simulink model "qhug_9"  (R2021a)
settings: Solver=ode45  StartTime=0.0  StopTime=1700  FixedStep=1  MaxStep=0.01  RelTol=1e-3
settings Model: Creator=daoist  LastModifiedBy=daoist

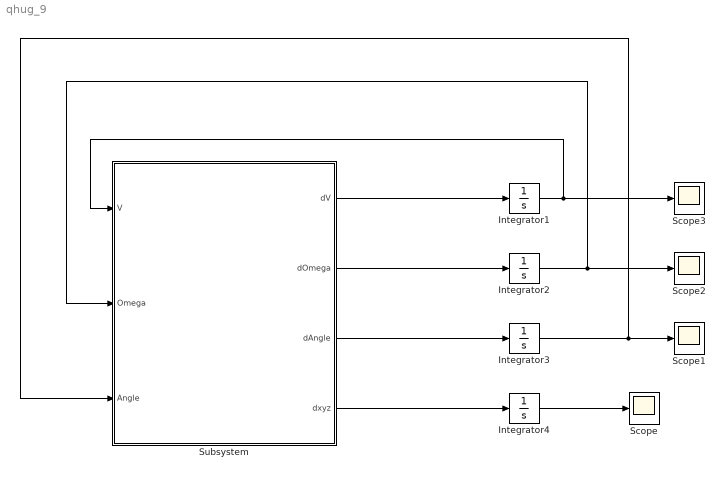
== system qhug_9 ==
  Integrator1 : Integrator  InitialCondition=[0.01 0 0 ]  LimitOutput=on  UpperSaturationLimit=[0.35 0.05 0.01]  LowerSaturationLimit=-[0.35 0.05 0.01]
  Integrator2 : Integrator
  Integrator3 : Integrator
  Integrator4 : Integrator
  Scope{,1..3} (4 alike) : Scope
  Subsystem : Subsystem
  wires:
  Subsystem/1(dV) -> Integrator1/1
  Subsystem/2(dOmega) -> Integrator2/1
  Subsystem/3(dAngle) -> Integrator3/1
  Subsystem/4(dxyz) -> Integrator4/1
  Integrator1/1 -> Scope3/1, Subsystem/1(V)
  Integrator2/1 -> Scope2/1, Subsystem/2(Omega)
  Integrator3/1 -> Scope1/1, Subsystem/3(Angle)
  Integrator4/1 -> Scope/1

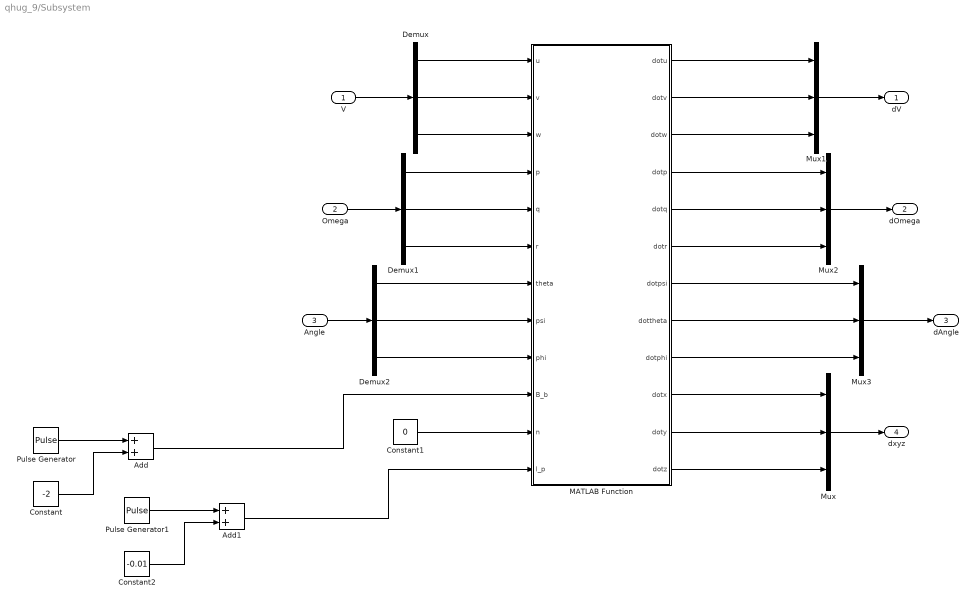
== system qhug_9/Subsystem ==
  V : Inport
  Omega : Inport  Port=2
  Angle : Inport  Port=3
  Add : Sum
  Add1 : Sum
  Constant : Constant  Value=-2
  Constant1 : Constant  Value=0
  Constant2 : Constant  Value=-0.01
  Demux : Demux  Outputs=3
  Demux1 : Demux  Outputs=3
  Demux2 : Demux  Outputs=3
  MATLAB Function : MATLAB Function  TreatAsAtomicUnit=on
  Mux{,1..3} (4 alike) : Mux  Inputs=3
  Pulse Generator : DiscretePulseGenerator  PulseType=Time based  Amplitude=4  Period=1700  PulseWidth=50
  Pulse Generator1 : DiscretePulseGenerator  PulseType=Time based  Amplitude=0.02  Period=1700  PulseWidth=50
  dV : Outport
  dOmega : Outport  Port=2
  dAngle : Outport  Port=3
  dxyz : Outport  Port=4
  wires:
  MATLAB Function/10(dotx) -> Mux/1
  MATLAB Function/11(doty) -> Mux/2
  MATLAB Function/12(dotz) -> Mux/3
  Mux/1 -> dxyz/1
  MATLAB Function/1(dotu) -> Mux1/1
  MATLAB Function/2(dotv) -> Mux1/2
  MATLAB Function/3(dotw) -> Mux1/3
  Mux1/1 -> dV/1
  MATLAB Function/4(dotp) -> Mux2/1
  MATLAB Function/5(dotq) -> Mux2/2
  MATLAB Function/6(dotr) -> Mux2/3
  Mux2/1 -> dOmega/1
  MATLAB Function/7(dotpsi) -> Mux3/1
  MATLAB Function/8(dottheta) -> Mux3/2
  MATLAB Function/9(dotphi) -> Mux3/3
  Mux3/1 -> dAngle/1
  Demux/1 -> MATLAB Function/1(u)
  Demux/2 -> MATLAB Function/2(v)
  Demux/3 -> MATLAB Function/3(w)
  V/1 -> Demux/1
  Demux1/1 -> MATLAB Function/4(p)
  Demux1/2 -> MATLAB Function/5(q)
  Demux1/3 -> MATLAB Function/6(r)
  Demux2/1 -> MATLAB Function/7(theta)
  Demux2/2 -> MATLAB Function/8(psi)
  Demux2/3 -> MATLAB Function/9(phi)
  Omega/1 -> Demux1/1
  Angle/1 -> Demux2/1
  Pulse Generator/1 -> Add/1
  Constant/1 -> Add/2
  Add/1 -> MATLAB Function/10(B_b)
  Constant1/1 -> MATLAB Function/11(n)
  Constant2/1 -> Add1/2
  Pulse Generator1/1 -> Add1/1
  Add1/1 -> MATLAB Function/12(l_p)

== matlab function qhug_9/Subsystem/MATLAB Function ==
  data: u input; dotu output; v input; w input; p input; q input; r input; theta input; psi input; phi input; B_b input; n input; l_p input; dotv output; dotw output; dotp output; dotq output; dotr output; dotpsi output; dottheta output; dotphi output; dotx output; doty output; dotz output
function [dotu,dotv,dotw,dotp,dotq,dotr,dotpsi,dottheta,dotphi,dotx,doty,dotz] = fcn(u,v,w,p,q,r,theta,psi,phi, B_b, n, l_p)
m = 69;
m_p = 18;
m_r = 18;
B_0=676.2;
A_d = 0.038;
L = 2.17;
l_b = 0.93;
e_r = 0.018;
x_G = 0;
y_G = 0.06;
z_G = 0;
J_bx = 0.54;
J_by = 19.75;
J_bz = 19.82;
K_t = 0.34;
K_q = 0.067;
t = 0.16;
d_p = 0.12;
rho = 1022;
g = 9.8;
rho_1 = 2700;
E = 69;
lambda_11 = 1.3;
lambda_22 = 79.66;
lambda_33 = 60.53;
lambda_44 = 0;
lambda_55 = 21.83;
lambda_66 = 23.56;
lambda_26 = -12.37;
lambda_35 = 19.35;
C_x0 =  -0.42;
C_ay = 0.5;
C_ry = -1.6;
C_bz  = 1.6;
C_qz = -0.17;
C_pz = 0;
T_bx = 0;
T_px = 0;
T_qx = 0;
T_by = 0.29;
T_qy = -0.35;
T_py = 0;
T_az = -0.41;
T_rz = -0.34;
G=m*g;

dotx = u * cos(theta) * cos(psi) + v*sin(psi)*sin(phi)-v*sin(theta)*cos(psi)*cos(phi)+...
    w*sin(psi)*cos(phi)+w*sin(theta)*cos(psi)*sin(phi);
doty = u*sin(theta)+v*cos(theta)*cos(phi)-w*cos(theta)*sin(phi);
dotz = -u*cos(theta)*sin(psi)+v*cos(psi)*sin(phi)+v*sin(theta)*sin(psi)*cos(phi)+...
    w*cos(psi)*cos(phi)-w*sin(theta)*sin(psi)*sin(phi);
dotpsi = q*cos(phi)/cos(theta) - r*sin(phi)/cos(theta);
dottheta = q*sin(phi)+r*cos(phi);
dotphi = p - q*cos(phi)*tan(theta)+r*sin(phi)*tan(theta);

A = [ m+lambda_11, 0,0,  0,0, -m*y_G;
    0, m+lambda_22,0,    0,0, lambda_26;
    0,0,m+lambda_33,   m*y_G, -lambda_35,0;
    0,0, m*y_G,   J_bx+lambda_44,0,0;
    0,0, lambda_35,  0,J_by+lambda_55,0;
    m*y_G, lambda_26, 0,   0,0, J_bz + lambda_66;];

V = sqrt(u^2 +v^2+w^2);
Alpha = atan(v/u);
Beta = atan(v/V);


p1 = p * L /V;
q1 = q * L /V;
r1 = r * L / V;

% B=[m*v*r-m*w*q-m*y_G*p*q-B_b*sin(theta)+(G-B_0)*sin(theta)+(1-t)*K_t*rho*n^2*d_p^4+0.5*rho*V^2*A_d*C_x0,...
%     m*w*p-m*u*r+m*y_G*(r^2+p^2)-B_b*cos(theta)*cos(phi)+(G-B_0)*cos(theta)*cos(phi)+0.5*rho*V^2*A_d*(C_ay*Alpha+C_ry*r1),...
%     m*u*q-m*v*p-m*y_G*r*q+B_b*cos(theta)*sin(phi)-(G-B_0)*cos(theta)*cos(phi)+0.5*rho*V^2*A_d*(C_bz*Beta+C_qz*q1+C_pz*p1),...
%     -m*y_G*(v*p-u*q)-(J_bz-J_by)*q*r-G*y_G*cos(theta)*sin(phi)+K_q*rho*n^2*d_p^5+m_r*g*e_r*((1-cos(psi))*cos(theta)*sin(phi)-sin(psi)*cos(theta)*cos(phi))+0.5*rho*V^2*A_d*L*(T_bx*Beta+T_px*p1+T_qx*q1),...
%     -(J_bx-J_bz)*r*p+(m_p*g*l_p-B_b*l_b)*cos(theta)*sin(phi)+m_r*g*e_r*sin(psi)*sin(theta)+0.5*rho*V^2*A_d*L*(T_by*Beta+T_qy*q1+T_py*p1),...
%     -m*y_G*(w*q-v*r)-(J_by-J_bx)*p*q+m_r*g*e_r*sin(theta)*(cos(psi)-1)+(B_b*l_b+m_p*g*l_p)*cos(theta)*cos(phi)+G*y_G*sin(theta)+0.5*rho*V^2*A_d*L*(T_az*Alpha+T_rz*r1);];

RB1 = m*v*r-m*w*q-m*y_G*p*q...
    -B_b*sin(theta)+(G-B_0)*sin(theta)+(1-t)*K_t*rho*n^2*d_p^4+0.5*rho*V^2*A_d*C_x0;
RB2 = m*w*p-m*u*r+m*y_G*(r^2+p^2)...
    -B_b*cos(theta)*cos(phi)+(G-B_0)*cos(theta)*cos(phi)+0.5*rho*V^2*A_d*(C_ay*Alpha+C_ry*r1);
RB3 = m*u*q-m*v*p-m*y_G*r*q...
    +B_b*cos(theta)*sin(phi)-(G-B_0)*cos(theta)*cos(phi)+0.5*rho*V^2*A_d*(C_bz*Beta+C_qz*q1+C_pz*p1);
RB4 = -m*y_G*(v*p-u*q)-(J_bz-J_by)*q*r-G*y_G*cos(theta)*sin(phi)...
    +K_q*rho*n^2*d_p^5+m_r*g*e_r*((1-cos(psi))*cos(theta)*sin(phi)-sin(psi)*cos(theta)*cos(phi))+0.5*rho*V^2*A_d*L*(T_bx*Beta+T_px*p1+T_qx*q1);
RB5 = -(J_bx-J_bz)*r*p...
    +(m_p*g*l_p-B_b*l_b)*cos(theta)*sin(phi)+m_r*g*e_r*sin(psi)*sin(theta)+0.5*rho*V^2*A_d*L*(T_by*Beta+T_qy*q1+T_py*p1);
RB6 = -m*y_G*(w*q-v*r)-(J_by-J_bx)*p*q+m_r*g*e_r*sin(theta)*(cos(psi)-1)...
    +(B_b*l_b+m_p*g*l_p)*cos(theta)*cos(phi)+G*y_G*sin(theta)+0.5*rho*V^2*A_d*L*(T_az*Alpha+T_rz*r1);
B = [RB1 RB2 RB3 RB4 RB5 RB6];

out = inv(A)*B';
dotu = out(1);
dotv = out(2);
dotw = out(3);
dotp = out(4);
dotq = out(5);
dotr = out(6);
